simulink model "EX7"  (R2020a)
settings: Solver=VariableStepAuto  StartTime=0.0  StopTime=10  MaxStep=0.001  RelTol=1e-3
values from neighbouring files (symbols this model uses):
  Kd = 3    [EX2.m]    (also in EX4.m = 1; EX8.m = 10; Untitled.m = 2)
libraries: cstblocks x5, simulink x2
settings Model: Creator=EREN  LastModifiedBy=EREN

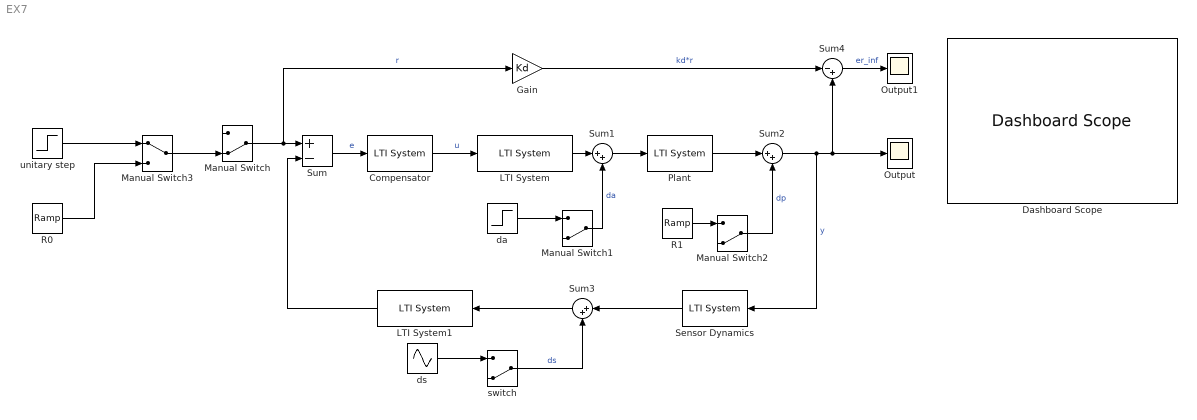
== system EX7 ==
  Compensator : cstblocks/LTI System  sys=Gc  IC=[]
  Dashboard Scope : DashboardScope
  Gain : Gain  Gain=Kd
  LTI System : cstblocks/LTI System  sys=Ga  IC=[]
  LTI System1 : cstblocks/LTI System  sys=Gf  IC=[]
  Manual Switch : ManualSwitch  CurrentSetting=0
  Manual Switch1 : ManualSwitch  CurrentSetting=0
  Manual Switch2 : ManualSwitch  CurrentSetting=0
  Manual Switch3 : ManualSwitch
  Output : Scope
  Output1 : Scope
  Plant : cstblocks/LTI System  sys=Gp  IC=[]
  R0 : simulink/Sources/Ramp  slope=1  start=0  InitialOutput=0
  R1 : simulink/Sources/Ramp  slope=8.5*10^-3  start=0  InitialOutput=0
  Sensor Dynamics : cstblocks/LTI System  sys=Gs  IC=[]
  Sum : Sum  Inputs=+-
  Sum1 : Sum  Inputs=|++
  Sum2 : Sum  Inputs=|++
  Sum3 : Sum  Inputs=|++
  Sum4 : Sum  Inputs=|-+
  da : Step  Time=0  After=2.5e-03  SampleTime=0
  ds : Sin  Amplitude=5e-02  Frequency=40  SampleTime=0
  switch : ManualSwitch  CurrentSetting=0
  unitary step : Step  Time=0  SampleTime=0
  wires:
  Manual Switch/1 -> Gain/1, Sum/1  "r"
  unitary step/1 -> Manual Switch3/1
  R0/1 -> Manual Switch3/2
  LTI System/1 -> Sum1/1
  da/1 -> Manual Switch1/1
  Manual Switch1/1 -> Sum1/2  "da"
  Sum/1 -> Compensator/1  "e"
  Compensator/1 -> LTI System/1  "u"
  Sum1/1 -> Plant/1
  Manual Switch2/1 -> Sum2/2  "dp"
  Plant/1 -> Sum2/1
  Sum2/1 -> Sensor Dynamics/1, Output/1, Sum4/2  "y"
  Sensor Dynamics/1 -> Sum3/1
  switch/1 -> Sum3/2  "ds"
  Sum3/1 -> LTI System1/1
  LTI System1/1 -> Sum/2
  Gain/1 -> Sum4/1  "kd*r"
  Sum4/1 -> Output1/1  "er_inf"
  ds/1 -> switch/1
  Manual Switch3/1 -> Manual Switch/2
  R1/1 -> Manual Switch2/1
